simulink model "gm_uz_sine_generator_16bit"  (R2023a)
settings: Solver=FixedStepDiscrete  StartTime=0.0  StopTime=50000/100e6  RelTol=1e-3
libraries: hdlsllib x8, embmathops x8, simulink x1
(part 1 of 2)
settings Model: Creator=ts  LastModifiedBy=ts
settings SolverCC: AlgebraicLoopSolver=TrustRegion
settings DataIOCC: LimitDataPoints=on  SaveOutput=off  SaveTime=off
settings OptimizationCC: BlockReduction=off  ConditionallyExecuteInputs=off  DefaultParameterBehavior=Inlined  LifeSpan=inf
settings DebuggingCC: AlgebraicLoopMsg=error  InheritedTsInSrcMsg=none  SingleTaskRateTransMsg=error  UnconnectedInputMsg=warning  UnconnectedOutputMsg=warning  UnconnectedLineMsg=warning  AllowSymbolicDim=off  StrictBusMsg=ErrorOnBusTreatedAsVector  SFUnexpectedBacktrackingDiag=warning  SFNoUnconditionalDefaultTransitionDiag=warning  SFExecutionAtInitializationDiag=none  ArithmeticOperatorsInVariantConditions=warning
settings HardwareCC: ProdBitPerPointer=32  ProdBitPerSizeT=32  ProdBitPerPtrDiffT=32  ProdLargestAtomicFloat=None  ProdIntDivRoundTo=Undefined  ProdEndianess=Unspecified  ProdWordSize=32  ProdHWDeviceType=ASIC/FPGA->ASIC/FPGA  ProdEqTarget=off
settings ModelReferenceCC: EnableRefExpFcnMdlSchedulingChecks=on
settings SFSimCC: SimUseLocalCustomCode=off  CustomCodeUndefinedFunction=UseInterfaceOnly
settings RTWCC: RTWUseLocalCustomCode=off
settings CodeAppCC: StateflowObjectComments=on
settings GRTTargetCC: TargetLangStandard=C89/C90 (ANSI)
settings ConfigComp: CovScope=ReferencedModels  CovMetricSettings=dw  CovSaveCumulativeToWorkspaceVar=on  CovSaveSingleToWorkspaceVar=on  CovExternalEMLEnable=off  CovSFcnEnable=off

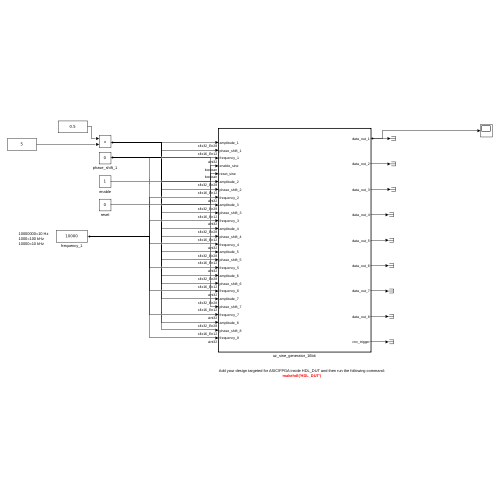
[thumbnail: Simulink's stored preview of the top-level diagram]
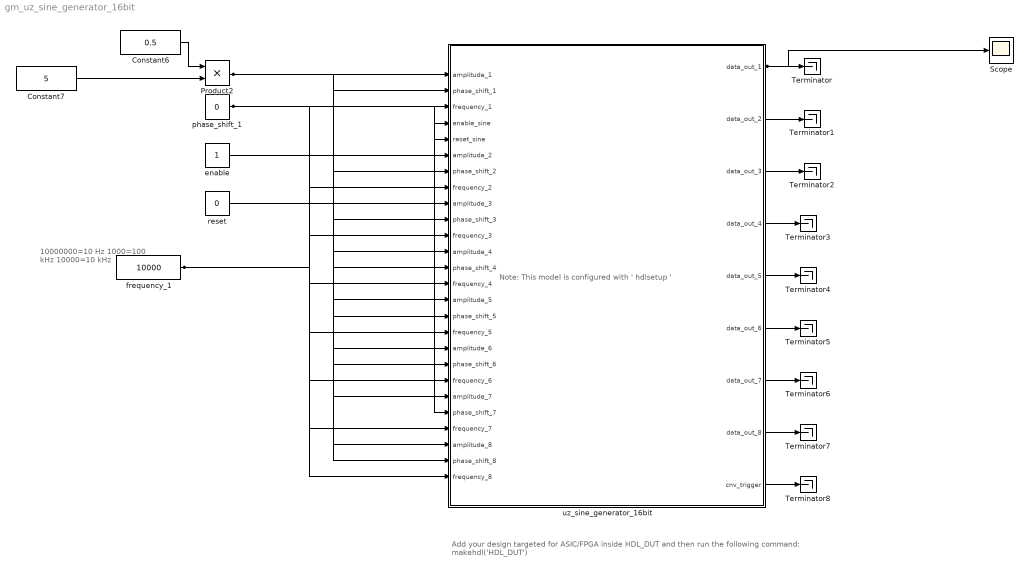
== system gm_uz_sine_generator_16bit ==
  note: 10000000=10 Hz
      | 1000=100 kHz
      | 10000=10 kHz
  note: Add your design targeted for ASIC/FPGA inside HDL_DUT and then run the following command:
      | makehdl('HDL_DUT')
  note: Note: This model is configured with ' hdlsetup '
  Constant6 : Constant  Value=0.5  SampleTime=-1
  Constant7 : Constant  Value=5  SampleTime=-1
  Product2 : Product  OutDataTypeStr=fixdt(1,32,28)
  Scope : Scope
  Terminator{,1..8} (9 alike) : Terminator
  enable : Constant  OutDataTypeStr=boolean  SampleTime=-1
  frequency_1 : Constant  Value=10000  OutDataTypeStr=uint32  SampleTime=1/100e6
  phase_shift_1 : Constant  Value=0  OutDataTypeStr=fixdt(1,16,12)  SampleTime=-1
  reset : Constant  Value=0  OutDataTypeStr=boolean  SampleTime=-1
  "uz_sine_generator_16bit " : Subsystem  TreatAsAtomicUnit=on
  wires:
  frequency_1/1 -> "uz_sine_generator_16bit "/8(frequency_2), "uz_sine_generator_16bit "/3(frequency_1), "uz_sine_generator_16bit "/11(frequency_3), "uz_sine_generator_16bit "/14(frequency_4), "uz_sine_generator_16bit "/17(frequency_5), "uz_sine_generator_16bit "/20(frequency_6), "uz_sine_generator_16bit "/23(frequency_7), "uz_sine_generator_16bit "/26(frequency_8)
  reset/1 -> "uz_sine_generator_16bit "/5(reset_sine)
  enable/1 -> "uz_sine_generator_16bit "/4(enable_sine)
  "uz_sine_generator_16bit "/9(cnv_trigger) -> Terminator8/1
  "uz_sine_generator_16bit "/8(data_out_8) -> Terminator7/1
  "uz_sine_generator_16bit "/7(data_out_7) -> Terminator6/1
  "uz_sine_generator_16bit "/6(data_out_6) -> Terminator5/1
  "uz_sine_generator_16bit "/5(data_out_5) -> Terminator4/1
  "uz_sine_generator_16bit "/4(data_out_4) -> Terminator3/1
  "uz_sine_generator_16bit "/3(data_out_3) -> Terminator2/1
  "uz_sine_generator_16bit "/2(data_out_2) -> Terminator1/1
  "uz_sine_generator_16bit "/1(data_out_1) -> Terminator/1, Scope/1
  phase_shift_1/1 -> "uz_sine_generator_16bit "/22(phase_shift_7), "uz_sine_generator_16bit "/19(phase_shift_6), "uz_sine_generator_16bit "/16(phase_shift_5), "uz_sine_generator_16bit "/10(phase_shift_3), "uz_sine_generator_16bit "/2(phase_shift_1), "uz_sine_generator_16bit "/7(phase_shift_2), "uz_sine_generator_16bit "/13(phase_shift_4), "uz_sine_generator_16bit "/25(phase_shift_8)
  Product2/1 -> "uz_sine_generator_16bit "/1(amplitude_1), "uz_sine_generator_16bit "/6(amplitude_2), "uz_sine_generator_16bit "/12(amplitude_4), "uz_sine_generator_16bit "/15(amplitude_5), "uz_sine_generator_16bit "/9(amplitude_3), "uz_sine_generator_16bit "/18(amplitude_6), "uz_sine_generator_16bit "/21(amplitude_7), "uz_sine_generator_16bit "/24(amplitude_8)
  Constant7/1 -> Product2/2
  Constant6/1 -> Product2/1

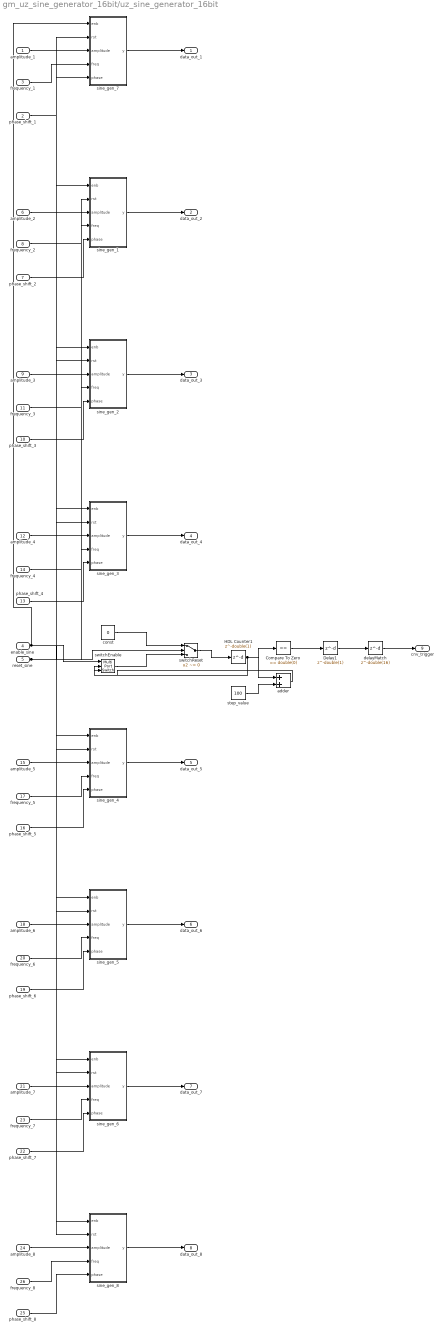
== system gm_uz_sine_generator_16bit/uz_sine_generator_16bit  ==
  amplitude_1 : Inport  OutDataTypeStr=fixdt(1, 32, 28)  PortDimensions=1  SampleTime=1e-08
  phase_shift_1 : Inport  Port=2  OutDataTypeStr=fixdt(1, 16, 12)  PortDimensions=1  SampleTime=1e-08
  frequency_1 : Inport  Port=3  OutDataTypeStr=uint32  PortDimensions=1  SampleTime=1e-08
  enable_sine : Inport  Port=4  OutDataTypeStr=boolean  PortDimensions=1  SampleTime=1e-08
  reset_sine : Inport  Port=5  OutDataTypeStr=boolean  PortDimensions=1  SampleTime=1e-08
  amplitude_2 : Inport  Port=6  OutDataTypeStr=fixdt(1, 32, 28)  PortDimensions=1  SampleTime=1e-08
  phase_shift_2 : Inport  Port=7  OutDataTypeStr=fixdt(1, 16, 12)  PortDimensions=1  SampleTime=1e-08
  frequency_2 : Inport  Port=8  OutDataTypeStr=uint32  PortDimensions=1  SampleTime=1e-08
  amplitude_3 : Inport  Port=9  OutDataTypeStr=fixdt(1, 32, 28)  PortDimensions=1  SampleTime=1e-08
  phase_shift_3 : Inport  Port=10  OutDataTypeStr=fixdt(1, 16, 12)  PortDimensions=1  SampleTime=1e-08
  frequency_3 : Inport  Port=11  OutDataTypeStr=uint32  PortDimensions=1  SampleTime=1e-08
  amplitude_4 : Inport  Port=12  OutDataTypeStr=fixdt(1, 32, 28)  PortDimensions=1  SampleTime=1e-08
  phase_shift_4 : Inport  Port=13  OutDataTypeStr=fixdt(1, 16, 12)  PortDimensions=1  SampleTime=1e-08
  frequency_4 : Inport  Port=14  OutDataTypeStr=uint32  PortDimensions=1  SampleTime=1e-08
  amplitude_5 : Inport  Port=15  OutDataTypeStr=fixdt(1, 32, 28)  PortDimensions=1  SampleTime=1e-08
  phase_shift_5 : Inport  Port=16  OutDataTypeStr=fixdt(1, 16, 12)  PortDimensions=1  SampleTime=1e-08
  frequency_5 : Inport  Port=17  OutDataTypeStr=uint32  PortDimensions=1  SampleTime=1e-08
  amplitude_6 : Inport  Port=18  OutDataTypeStr=fixdt(1, 32, 28)  PortDimensions=1  SampleTime=1e-08
  phase_shift_6 : Inport  Port=19  OutDataTypeStr=fixdt(1, 16, 12)  PortDimensions=1  SampleTime=1e-08
  frequency_6 : Inport  Port=20  OutDataTypeStr=uint32  PortDimensions=1  SampleTime=1e-08
  amplitude_7 : Inport  Port=21  OutDataTypeStr=fixdt(1, 32, 28)  PortDimensions=1  SampleTime=1e-08
  phase_shift_7 : Inport  Port=22  OutDataTypeStr=fixdt(1, 16, 12)  PortDimensions=1  SampleTime=1e-08
  frequency_7 : Inport  Port=23  OutDataTypeStr=uint32  PortDimensions=1  SampleTime=1e-08
  amplitude_8 : Inport  Port=24  OutDataTypeStr=fixdt(1, 32, 28)  PortDimensions=1  SampleTime=1e-08
  phase_shift_8 : Inport  Port=25  OutDataTypeStr=fixdt(1, 16, 12)  PortDimensions=1  SampleTime=1e-08
  frequency_8 : Inport  Port=26  OutDataTypeStr=uint32  PortDimensions=1  SampleTime=1e-08
  Compare To Zero : simulink/Logic and Bit Operations/Compare To Constant  relop===  const=double(0)  OutDataTypeStr=boolean
  Delay1 : Delay  DelayLength=double(1)  InitialCondition=0  SampleTime=1e-08
  HDL Counter1 : Delay  DelayLength=double(1)  InitialCondition=0  SampleTime=1e-08
  adder : Sum  AccumDataTypeStr=uint8  OutDataTypeStr=uint8  SampleTime=1e-08
  const : Constant  Value=0  VectorParams1D=off  OutDataTypeStr=uint8  SampleTime=1e-08
  delayMatch : Delay  DelayLength=double(16)  InitialCondition=0  SampleTime=1e-08
  sine_gen_1 : Subsystem
  sine_gen_2 : Subsystem
  sine_gen_3 : Subsystem
  sine_gen_4 : Subsystem
  sine_gen_5 : Subsystem
  sine_gen_6 : Subsystem
  sine_gen_7 : Subsystem
  sine_gen_8 : Subsystem
  step_value : Constant  Value=100  VectorParams1D=off  OutDataTypeStr=uint8  SampleTime=1e-08
  switchEnable : MultiPortSwitch  DataPortOrder=Zero-based contiguous  Inputs=2  DiagnosticForDefault=None  zeroidx=on  OutDataTypeStr=uint8  SampleTime=1e-08  SaturateOnIntegerOverflow=off  InputSameDT=off
  switchReset : Switch  Criteria=u2 ~= 0  Threshold=double(0)  OutDataTypeStr=uint8  SampleTime=1e-08  SaturateOnIntegerOverflow=off  InputSameDT=off
  data_out_1 : Outport  SampleTime=1e-08  VectorParamsAs1DForOutWhenUnconnected=off
  data_out_2 : Outport  Port=2  SampleTime=1e-08  VectorParamsAs1DForOutWhenUnconnected=off
  data_out_3 : Outport  Port=3  SampleTime=1e-08  VectorParamsAs1DForOutWhenUnconnected=off
  data_out_4 : Outport  Port=4  SampleTime=1e-08  VectorParamsAs1DForOutWhenUnconnected=off
  data_out_5 : Outport  Port=5  SampleTime=1e-08  VectorParamsAs1DForOutWhenUnconnected=off
  data_out_6 : Outport  Port=6  SampleTime=1e-08  VectorParamsAs1DForOutWhenUnconnected=off
  data_out_7 : Outport  Port=7  SampleTime=1e-08  VectorParamsAs1DForOutWhenUnconnected=off
  data_out_8 : Outport  Port=8  SampleTime=1e-08  VectorParamsAs1DForOutWhenUnconnected=off
  cnv_trigger : Outport  Port=9  SampleTime=1e-08  VectorParamsAs1DForOutWhenUnconnected=off
  wires:
  amplitude_1/1 -> sine_gen_7/3(amplitude)
  phase_shift_1/1 -> sine_gen_7/5(phase)
  frequency_1/1 -> sine_gen_7/4(freq)
  enable_sine/1 -> sine_gen_7/1(enb), sine_gen_1/1(enb), sine_gen_2/1(enb), sine_gen_3/1(enb), sine_gen_4/1(enb), sine_gen_5/1(enb), sine_gen_8/1(enb), sine_gen_6/1(enb), switchEnable/1
  reset_sine/1 -> sine_gen_1/2(rst), sine_gen_2/2(rst), sine_gen_3/2(rst), sine_gen_4/2(rst), sine_gen_5/2(rst), sine_gen_8/2(rst), sine_gen_6/2(rst), sine_gen_7/2(rst), switchReset/2
  amplitude_2/1 -> sine_gen_1/3(amplitude)
  phase_shift_2/1 -> sine_gen_1/5(phase)
  frequency_2/1 -> sine_gen_1/4(freq)
  amplitude_3/1 -> sine_gen_2/3(amplitude)
  phase_shift_3/1 -> sine_gen_2/5(phase)
  frequency_3/1 -> sine_gen_2/4(freq)
  amplitude_4/1 -> sine_gen_3/3(amplitude)
  phase_shift_4/1 -> sine_gen_3/5(phase)
  frequency_4/1 -> sine_gen_3/4(freq)
  amplitude_5/1 -> sine_gen_4/3(amplitude)
  phase_shift_5/1 -> sine_gen_4/5(phase)
  frequency_5/1 -> sine_gen_4/4(freq)
  amplitude_6/1 -> sine_gen_5/3(amplitude)
  phase_shift_6/1 -> sine_gen_5/5(phase)
  frequency_6/1 -> sine_gen_5/4(freq)
  amplitude_7/1 -> sine_gen_6/3(amplitude)
  phase_shift_7/1 -> sine_gen_6/5(phase)
  frequency_7/1 -> sine_gen_6/4(freq)
  amplitude_8/1 -> sine_gen_8/3(amplitude)
  phase_shift_8/1 -> sine_gen_8/5(phase)
  frequency_8/1 -> sine_gen_8/4(freq)
  Compare To Zero/1 -> Delay1/1
  delayMatch/1 -> cnv_trigger/1
  sine_gen_1/1(y) -> data_out_2/1
  sine_gen_7/1(y) -> data_out_1/1
  sine_gen_2/1(y) -> data_out_3/1
  sine_gen_3/1(y) -> data_out_4/1
  sine_gen_4/1(y) -> data_out_5/1
  sine_gen_5/1(y) -> data_out_6/1
  sine_gen_6/1(y) -> data_out_7/1
  sine_gen_8/1(y) -> data_out_8/1
  HDL Counter1/1 -> Compare To Zero/1, adder/1, switchEnable/2
  const/1 -> switchReset/1
  step_value/1 -> adder/2
  Delay1/1 -> delayMatch/1
  switchReset/1 -> HDL Counter1/1
  adder/1 -> switchEnable/3
  switchEnable/1 -> switchReset/3

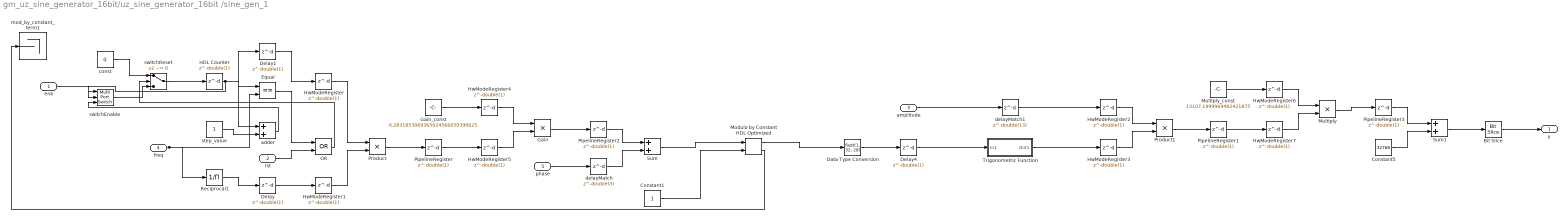
== system gm_uz_sine_generator_16bit/uz_sine_generator_16bit /sine_gen_1 ==
  enb : Inport  OutDataTypeStr=boolean  PortDimensions=1  SampleTime=1e-08
  rst : Inport  Port=2  OutDataTypeStr=boolean  PortDimensions=1  SampleTime=1e-08
  amplitude : Inport  Port=3  OutDataTypeStr=fixdt(1, 32, 28)  PortDimensions=1  SampleTime=1e-08
  freq : Inport  Port=4  OutDataTypeStr=uint32  PortDimensions=1  SampleTime=1e-08
  phase : Inport  Port=5  OutDataTypeStr=fixdt(1, 16, 12)  PortDimensions=1  SampleTime=1e-08
  Bit Slice : hdlsllib/Logic and Bit Operations/Bit Slice  lidx=double(15)  ridx=double(0)
  Constant1 : Constant  OutDataTypeStr=boolean  SampleTime=1e-08
  Constant5 : Constant  Value=32768  OutDataTypeStr=int32  SampleTime=1e-08
  Data Type Conversion : DataTypeConversion  OutDataTypeStr=fixdt(1, 32, 28)  SampleTime=1e-08  SaturateOnIntegerOverflow=off  RndMeth=Floor
  Delay : Delay  DelayLength=double(1)  InitialCondition=0  SampleTime=1e-08
  Delay1 : Delay  DelayLength=double(1)  InitialCondition=0  SampleTime=1e-08
  Delay4 : Delay  DelayLength=double(1)  InitialCondition=0  SampleTime=1e-08
  Equal : RelationalOperator  Operator===  OutDataTypeStr=boolean  SampleTime=1e-08  InputSameDT=off
  Gain : Product  Inputs=**  OutDataTypeStr=fixdt(1, 32, 28)  SampleTime=1e-08
  Gain_const : Constant  Value=6.2831853069365024566650390625  OutDataTypeStr=fixdt(0, 32, 29)  SampleTime=1e-08
  HDL Counter : Delay  DelayLength=double(1)  InitialCondition=0  SampleTime=1e-08
  HwModeRegister{,1..7} (8 alike) : Delay  DelayLength=double(1)  InitialCondition=0  SampleTime=1e-08
  Modulo by Constant HDL Optimized : embmathops/Modulo by Constant HDL Optimized  Denominator=2*pi  SimulateUsing=Code generation
      settings: LibrarySourceBlock=|
      | embeddedMatrixLib/Math Operations/Modulo by Constant
      | HDL Optimized
  Multiply : Product  Inputs=**  OutDataTypeStr=int32  SampleTime=1e-08
  Multiply_const : Constant  Value=13107.1999969482421875  OutDataTypeStr=fixdt(1, 32, 17)  SampleTime=1e-08
  OR : Logic  Operator=OR  AllPortsSameDT=off  OutDataTypeStr=boolean  SampleTime=1e-08
  PipelineRegister{,1..3} (4 alike) : Delay  DelayLength=double(1)  InitialCondition=0  SampleTime=1e-08
  Product : Product  Inputs=**  OutDataTypeStr=fixdt(0, 32, 29)  SampleTime=1e-08
  Product1 : Product  Inputs=**  OutDataTypeStr=fixdt(1, 32, 28)  SampleTime=1e-08
  Reciprocal1 : Product  Inputs=/  OutDataTypeStr=fixdt(0, 32, 31)  RndMeth=Zero  SaturateOnIntegerOverflow=on  SampleTime=1e-08
  Sum : Sum  AccumDataTypeStr=fixdt(1, 33, 28)  OutDataTypeStr=fixdt(1, 33, 28)  SampleTime=1e-08
  Sum1 : Sum  AccumDataTypeStr=int32  OutDataTypeStr=int32  SampleTime=1e-08
  Trigonometric Function : Subsystem
  adder : Sum  AccumDataTypeStr=uint32  OutDataTypeStr=uint32  SampleTime=1e-08
  const : Constant  Value=0  VectorParams1D=off  OutDataTypeStr=uint32  SampleTime=1e-08
  delayMatch : Delay  DelayLength=double(3)  InitialCondition=0  SampleTime=1e-08
  delayMatch1 : Delay  DelayLength=double(13)  InitialCondition=0  SampleTime=1e-08
  mod_by_constant_term1 : Terminator
  step_value : Constant  VectorParams1D=off  OutDataTypeStr=uint32  SampleTime=1e-08
  switchEnable : MultiPortSwitch  DataPortOrder=Zero-based contiguous  Inputs=2  DiagnosticForDefault=None  zeroidx=on  OutDataTypeStr=uint32  SampleTime=1e-08  SaturateOnIntegerOverflow=off  InputSameDT=off
  switchReset : Switch  Criteria=u2 ~= 0  Threshold=double(0)  OutDataTypeStr=uint32  SampleTime=1e-08  SaturateOnIntegerOverflow=off  InputSameDT=off
  y : Outport  SampleTime=1e-08
  wires:
  delayMatch1/1 -> HwModeRegister2/1
  delayMatch/1 -> Sum/2
  Bit Slice/1 -> y/1
  Constant1/1 -> Modulo by Constant HDL Optimized/2
  Constant5/1 -> Sum1/2
  Data Type Conversion/1 -> Delay4/1
  Delay/1 -> HwModeRegister1/1
  Delay1/1 -> HwModeRegister/1
  Sum/1 -> Modulo by Constant HDL Optimized/1
  Delay4/1 -> Trigonometric Function/1(In1)
  Trigonometric Function/1(Out1) -> HwModeRegister3/1
  PipelineRegister2/1 -> Sum/1
  Modulo by Constant HDL Optimized/1 -> Data Type Conversion/1
  Modulo by Constant HDL Optimized/2 -> mod_by_constant_term1/1
  PipelineRegister3/1 -> Sum1/1
  PipelineRegister/1 -> HwModeRegister5/1
  PipelineRegister1/1 -> HwModeRegister7/1
  Reciprocal1/1 -> Delay/1
  Sum1/1 -> Bit Slice/1
  HDL Counter/1 -> Delay1/1, Equal/1, adder/1, switchEnable/2
  const/1 -> switchReset/1
  step_value/1 -> adder/2
  Gain_const/1 -> HwModeRegister4/1
  Multiply_const/1 -> HwModeRegister6/1
  enb/1 -> switchEnable/1
  rst/1 -> OR/2
  amplitude/1 -> delayMatch1/1
  freq/1 -> Reciprocal1/1, Equal/2
  phase/1 -> delayMatch/1
  switchReset/1 -> HDL Counter/1
  adder/1 -> switchEnable/3
  switchEnable/1 -> switchReset/3
  Equal/1 -> OR/1
  OR/1 -> switchReset/2
  Product/1 -> PipelineRegister/1
  HwModeRegister/1 -> Product/1
  HwModeRegister1/1 -> Product/2
  Product1/1 -> PipelineRegister1/1
  HwModeRegister2/1 -> Product1/1
  HwModeRegister3/1 -> Product1/2
  Gain/1 -> PipelineRegister2/1
  HwModeRegister4/1 -> Gain/1
  HwModeRegister5/1 -> Gain/2
  Multiply/1 -> PipelineRegister3/1
  HwModeRegister6/1 -> Multiply/1
  HwModeRegister7/1 -> Multiply/2

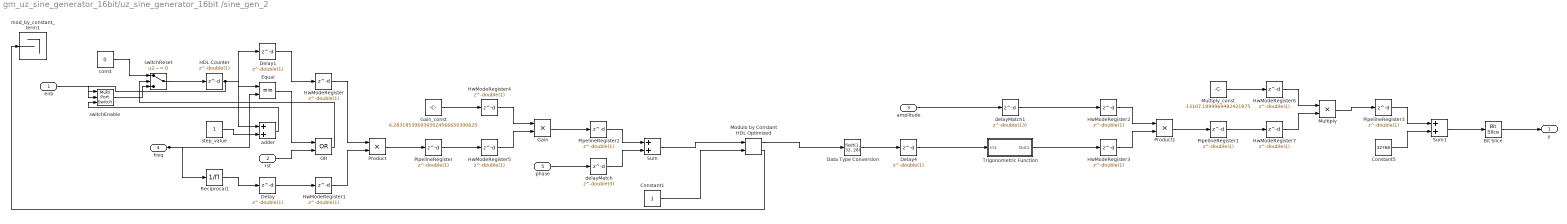
== system gm_uz_sine_generator_16bit/uz_sine_generator_16bit /sine_gen_2 ==
  enb : Inport  OutDataTypeStr=boolean  PortDimensions=1  SampleTime=1e-08
  rst : Inport  Port=2  OutDataTypeStr=boolean  PortDimensions=1  SampleTime=1e-08
  amplitude : Inport  Port=3  OutDataTypeStr=fixdt(1, 32, 28)  PortDimensions=1  SampleTime=1e-08
  freq : Inport  Port=4  OutDataTypeStr=uint32  PortDimensions=1  SampleTime=1e-08
  phase : Inport  Port=5  OutDataTypeStr=fixdt(1, 16, 12)  PortDimensions=1  SampleTime=1e-08
  Bit Slice : hdlsllib/Logic and Bit Operations/Bit Slice  lidx=double(15)  ridx=double(0)
  Constant1 : Constant  OutDataTypeStr=boolean  SampleTime=1e-08
  Constant5 : Constant  Value=32768  OutDataTypeStr=int32  SampleTime=1e-08
  Data Type Conversion : DataTypeConversion  OutDataTypeStr=fixdt(1, 32, 28)  SampleTime=1e-08  SaturateOnIntegerOverflow=off  RndMeth=Floor
  Delay : Delay  DelayLength=double(1)  InitialCondition=0  SampleTime=1e-08
  Delay1 : Delay  DelayLength=double(1)  InitialCondition=0  SampleTime=1e-08
  Delay4 : Delay  DelayLength=double(1)  InitialCondition=0  SampleTime=1e-08
  Equal : RelationalOperator  Operator===  OutDataTypeStr=boolean  SampleTime=1e-08  InputSameDT=off
  Gain : Product  Inputs=**  OutDataTypeStr=fixdt(1, 32, 28)  SampleTime=1e-08
  Gain_const : Constant  Value=6.2831853069365024566650390625  OutDataTypeStr=fixdt(0, 32, 29)  SampleTime=1e-08
  HDL Counter : Delay  DelayLength=double(1)  InitialCondition=0  SampleTime=1e-08
  HwModeRegister{,1..7} (8 alike) : Delay  DelayLength=double(1)  InitialCondition=0  SampleTime=1e-08
  Modulo by Constant HDL Optimized : embmathops/Modulo by Constant HDL Optimized  Denominator=2*pi  SimulateUsing=Code generation
      settings: LibrarySourceBlock=|
      | embeddedMatrixLib/Math Operations/Modulo by Constant
      | HDL Optimized
  Multiply : Product  Inputs=**  OutDataTypeStr=int32  SampleTime=1e-08
  Multiply_const : Constant  Value=13107.1999969482421875  OutDataTypeStr=fixdt(1, 32, 17)  SampleTime=1e-08
  OR : Logic  Operator=OR  AllPortsSameDT=off  OutDataTypeStr=boolean  SampleTime=1e-08
  PipelineRegister{,1..3} (4 alike) : Delay  DelayLength=double(1)  InitialCondition=0  SampleTime=1e-08
  Product : Product  Inputs=**  OutDataTypeStr=fixdt(0, 32, 29)  SampleTime=1e-08
  Product1 : Product  Inputs=**  OutDataTypeStr=fixdt(1, 32, 28)  SampleTime=1e-08
  Reciprocal1 : Product  Inputs=/  OutDataTypeStr=fixdt(0, 32, 31)  RndMeth=Zero  SaturateOnIntegerOverflow=on  SampleTime=1e-08
  Sum : Sum  AccumDataTypeStr=fixdt(1, 33, 28)  OutDataTypeStr=fixdt(1, 33, 28)  SampleTime=1e-08
  Sum1 : Sum  AccumDataTypeStr=int32  OutDataTypeStr=int32  SampleTime=1e-08
  Trigonometric Function : Subsystem
  adder : Sum  AccumDataTypeStr=uint32  OutDataTypeStr=uint32  SampleTime=1e-08
  const : Constant  Value=0  VectorParams1D=off  OutDataTypeStr=uint32  SampleTime=1e-08
  delayMatch : Delay  DelayLength=double(3)  InitialCondition=0  SampleTime=1e-08
  delayMatch1 : Delay  DelayLength=double(13)  InitialCondition=0  SampleTime=1e-08
  mod_by_constant_term1 : Terminator
  step_value : Constant  VectorParams1D=off  OutDataTypeStr=uint32  SampleTime=1e-08
  switchEnable : MultiPortSwitch  DataPortOrder=Zero-based contiguous  Inputs=2  DiagnosticForDefault=None  zeroidx=on  OutDataTypeStr=uint32  SampleTime=1e-08  SaturateOnIntegerOverflow=off  InputSameDT=off
  switchReset : Switch  Criteria=u2 ~= 0  Threshold=double(0)  OutDataTypeStr=uint32  SampleTime=1e-08  SaturateOnIntegerOverflow=off  InputSameDT=off
  y : Outport  SampleTime=1e-08
  wires:
  delayMatch1/1 -> HwModeRegister2/1
  delayMatch/1 -> Sum/2
  Bit Slice/1 -> y/1
  Constant1/1 -> Modulo by Constant HDL Optimized/2
  Constant5/1 -> Sum1/2
  Data Type Conversion/1 -> Delay4/1
  Delay/1 -> HwModeRegister1/1
  Delay1/1 -> HwModeRegister/1
  Sum/1 -> Modulo by Constant HDL Optimized/1
  Delay4/1 -> Trigonometric Function/1(In1)
  Trigonometric Function/1(Out1) -> HwModeRegister3/1
  PipelineRegister2/1 -> Sum/1
  Modulo by Constant HDL Optimized/1 -> Data Type Conversion/1
  Modulo by Constant HDL Optimized/2 -> mod_by_constant_term1/1
  PipelineRegister3/1 -> Sum1/1
  PipelineRegister/1 -> HwModeRegister5/1
  PipelineRegister1/1 -> HwModeRegister7/1
  Reciprocal1/1 -> Delay/1
  Sum1/1 -> Bit Slice/1
  HDL Counter/1 -> Delay1/1, Equal/1, adder/1, switchEnable/2
  const/1 -> switchReset/1
  step_value/1 -> adder/2
  Gain_const/1 -> HwModeRegister4/1
  Multiply_const/1 -> HwModeRegister6/1
  enb/1 -> switchEnable/1
  rst/1 -> OR/2
  amplitude/1 -> delayMatch1/1
  freq/1 -> Reciprocal1/1, Equal/2
  phase/1 -> delayMatch/1
  switchReset/1 -> HDL Counter/1
  adder/1 -> switchEnable/3
  switchEnable/1 -> switchReset/3
  Equal/1 -> OR/1
  OR/1 -> switchReset/2
  Product/1 -> PipelineRegister/1
  HwModeRegister/1 -> Product/1
  HwModeRegister1/1 -> Product/2
  Product1/1 -> PipelineRegister1/1
  HwModeRegister2/1 -> Product1/1
  HwModeRegister3/1 -> Product1/2
  Gain/1 -> PipelineRegister2/1
  HwModeRegister4/1 -> Gain/1
  HwModeRegister5/1 -> Gain/2
  Multiply/1 -> PipelineRegister3/1
  HwModeRegister6/1 -> Multiply/1
  HwModeRegister7/1 -> Multiply/2

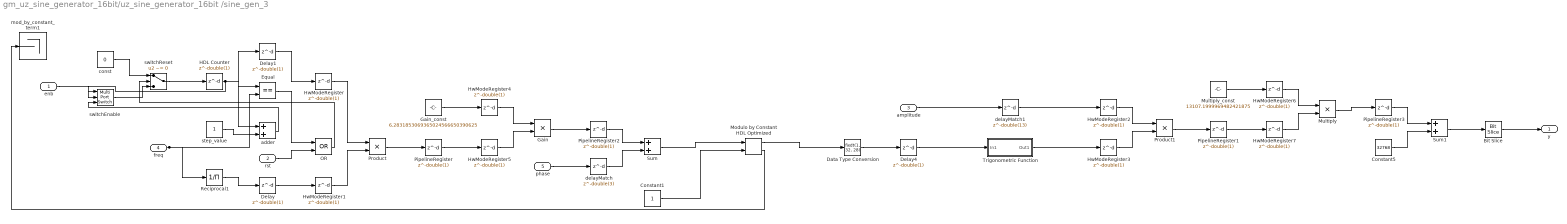
== system gm_uz_sine_generator_16bit/uz_sine_generator_16bit /sine_gen_3 ==
  enb : Inport  OutDataTypeStr=boolean  PortDimensions=1  SampleTime=1e-08
  rst : Inport  Port=2  OutDataTypeStr=boolean  PortDimensions=1  SampleTime=1e-08
  amplitude : Inport  Port=3  OutDataTypeStr=fixdt(1, 32, 28)  PortDimensions=1  SampleTime=1e-08
  freq : Inport  Port=4  OutDataTypeStr=uint32  PortDimensions=1  SampleTime=1e-08
  phase : Inport  Port=5  OutDataTypeStr=fixdt(1, 16, 12)  PortDimensions=1  SampleTime=1e-08
  Bit Slice : hdlsllib/Logic and Bit Operations/Bit Slice  lidx=double(15)  ridx=double(0)
  Constant1 : Constant  OutDataTypeStr=boolean  SampleTime=1e-08
  Constant5 : Constant  Value=32768  OutDataTypeStr=int32  SampleTime=1e-08
  Data Type Conversion : DataTypeConversion  OutDataTypeStr=fixdt(1, 32, 28)  SampleTime=1e-08  SaturateOnIntegerOverflow=off  RndMeth=Floor
  Delay : Delay  DelayLength=double(1)  InitialCondition=0  SampleTime=1e-08
  Delay1 : Delay  DelayLength=double(1)  InitialCondition=0  SampleTime=1e-08
  Delay4 : Delay  DelayLength=double(1)  InitialCondition=0  SampleTime=1e-08
  Equal : RelationalOperator  Operator===  OutDataTypeStr=boolean  SampleTime=1e-08  InputSameDT=off
  Gain : Product  Inputs=**  OutDataTypeStr=fixdt(1, 32, 28)  SampleTime=1e-08
  Gain_const : Constant  Value=6.2831853069365024566650390625  OutDataTypeStr=fixdt(0, 32, 29)  SampleTime=1e-08
  HDL Counter : Delay  DelayLength=double(1)  InitialCondition=0  SampleTime=1e-08
  HwModeRegister{,1..7} (8 alike) : Delay  DelayLength=double(1)  InitialCondition=0  SampleTime=1e-08
  Modulo by Constant HDL Optimized : embmathops/Modulo by Constant HDL Optimized  Denominator=2*pi  SimulateUsing=Code generation
      settings: LibrarySourceBlock=|
      | embeddedMatrixLib/Math Operations/Modulo by Constant
      | HDL Optimized
  Multiply : Product  Inputs=**  OutDataTypeStr=int32  SampleTime=1e-08
  Multiply_const : Constant  Value=13107.1999969482421875  OutDataTypeStr=fixdt(1, 32, 17)  SampleTime=1e-08
  OR : Logic  Operator=OR  AllPortsSameDT=off  OutDataTypeStr=boolean  SampleTime=1e-08
  PipelineRegister{,1..3} (4 alike) : Delay  DelayLength=double(1)  InitialCondition=0  SampleTime=1e-08
  Product : Product  Inputs=**  OutDataTypeStr=fixdt(0, 32, 29)  SampleTime=1e-08
  Product1 : Product  Inputs=**  OutDataTypeStr=fixdt(1, 32, 28)  SampleTime=1e-08
  Reciprocal1 : Product  Inputs=/  OutDataTypeStr=fixdt(0, 32, 31)  RndMeth=Zero  SaturateOnIntegerOverflow=on  SampleTime=1e-08
  Sum : Sum  AccumDataTypeStr=fixdt(1, 33, 28)  OutDataTypeStr=fixdt(1, 33, 28)  SampleTime=1e-08
  Sum1 : Sum  AccumDataTypeStr=int32  OutDataTypeStr=int32  SampleTime=1e-08
  Trigonometric Function : Subsystem
  adder : Sum  AccumDataTypeStr=uint32  OutDataTypeStr=uint32  SampleTime=1e-08
  const : Constant  Value=0  VectorParams1D=off  OutDataTypeStr=uint32  SampleTime=1e-08
  delayMatch : Delay  DelayLength=double(3)  InitialCondition=0  SampleTime=1e-08
  delayMatch1 : Delay  DelayLength=double(13)  InitialCondition=0  SampleTime=1e-08
  mod_by_constant_term1 : Terminator
  step_value : Constant  VectorParams1D=off  OutDataTypeStr=uint32  SampleTime=1e-08
  switchEnable : MultiPortSwitch  DataPortOrder=Zero-based contiguous  Inputs=2  DiagnosticForDefault=None  zeroidx=on  OutDataTypeStr=uint32  SampleTime=1e-08  SaturateOnIntegerOverflow=off  InputSameDT=off
  switchReset : Switch  Criteria=u2 ~= 0  Threshold=double(0)  OutDataTypeStr=uint32  SampleTime=1e-08  SaturateOnIntegerOverflow=off  InputSameDT=off
  y : Outport  SampleTime=1e-08
  wires:
  delayMatch1/1 -> HwModeRegister2/1
  delayMatch/1 -> Sum/2
  Bit Slice/1 -> y/1
  Constant1/1 -> Modulo by Constant HDL Optimized/2
  Constant5/1 -> Sum1/2
  Data Type Conversion/1 -> Delay4/1
  Delay/1 -> HwModeRegister1/1
  Delay1/1 -> HwModeRegister/1
  Sum/1 -> Modulo by Constant HDL Optimized/1
  Delay4/1 -> Trigonometric Function/1(In1)
  Trigonometric Function/1(Out1) -> HwModeRegister3/1
  PipelineRegister2/1 -> Sum/1
  Modulo by Constant HDL Optimized/1 -> Data Type Conversion/1
  Modulo by Constant HDL Optimized/2 -> mod_by_constant_term1/1
  PipelineRegister3/1 -> Sum1/1
  PipelineRegister/1 -> HwModeRegister5/1
  PipelineRegister1/1 -> HwModeRegister7/1
  Reciprocal1/1 -> Delay/1
  Sum1/1 -> Bit Slice/1
  HDL Counter/1 -> Delay1/1, Equal/1, adder/1, switchEnable/2
  const/1 -> switchReset/1
  step_value/1 -> adder/2
  Gain_const/1 -> HwModeRegister4/1
  Multiply_const/1 -> HwModeRegister6/1
  enb/1 -> switchEnable/1
  rst/1 -> OR/2
  amplitude/1 -> delayMatch1/1
  freq/1 -> Reciprocal1/1, Equal/2
  phase/1 -> delayMatch/1
  switchReset/1 -> HDL Counter/1
  adder/1 -> switchEnable/3
  switchEnable/1 -> switchReset/3
  Equal/1 -> OR/1
  OR/1 -> switchReset/2
  Product/1 -> PipelineRegister/1
  HwModeRegister/1 -> Product/1
  HwModeRegister1/1 -> Product/2
  Product1/1 -> PipelineRegister1/1
  HwModeRegister2/1 -> Product1/1
  HwModeRegister3/1 -> Product1/2
  Gain/1 -> PipelineRegister2/1
  HwModeRegister4/1 -> Gain/1
  HwModeRegister5/1 -> Gain/2
  Multiply/1 -> PipelineRegister3/1
  HwModeRegister6/1 -> Multiply/1
  HwModeRegister7/1 -> Multiply/2

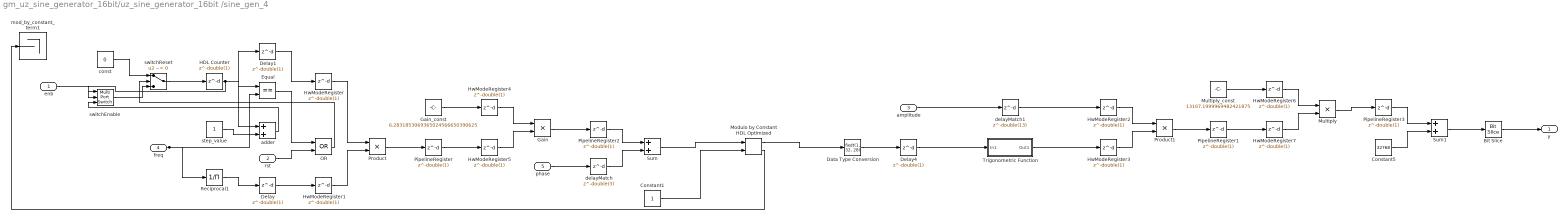
== system gm_uz_sine_generator_16bit/uz_sine_generator_16bit /sine_gen_4 ==
  enb : Inport  OutDataTypeStr=boolean  PortDimensions=1  SampleTime=1e-08
  rst : Inport  Port=2  OutDataTypeStr=boolean  PortDimensions=1  SampleTime=1e-08
  amplitude : Inport  Port=3  OutDataTypeStr=fixdt(1, 32, 28)  PortDimensions=1  SampleTime=1e-08
  freq : Inport  Port=4  OutDataTypeStr=uint32  PortDimensions=1  SampleTime=1e-08
  phase : Inport  Port=5  OutDataTypeStr=fixdt(1, 16, 12)  PortDimensions=1  SampleTime=1e-08
  Bit Slice : hdlsllib/Logic and Bit Operations/Bit Slice  lidx=double(15)  ridx=double(0)
  Constant1 : Constant  OutDataTypeStr=boolean  SampleTime=1e-08
  Constant5 : Constant  Value=32768  OutDataTypeStr=int32  SampleTime=1e-08
  Data Type Conversion : DataTypeConversion  OutDataTypeStr=fixdt(1, 32, 28)  SampleTime=1e-08  SaturateOnIntegerOverflow=off  RndMeth=Floor
  Delay : Delay  DelayLength=double(1)  InitialCondition=0  SampleTime=1e-08
  Delay1 : Delay  DelayLength=double(1)  InitialCondition=0  SampleTime=1e-08
  Delay4 : Delay  DelayLength=double(1)  InitialCondition=0  SampleTime=1e-08
  Equal : RelationalOperator  Operator===  OutDataTypeStr=boolean  SampleTime=1e-08  InputSameDT=off
  Gain : Product  Inputs=**  OutDataTypeStr=fixdt(1, 32, 28)  SampleTime=1e-08
  Gain_const : Constant  Value=6.2831853069365024566650390625  OutDataTypeStr=fixdt(0, 32, 29)  SampleTime=1e-08
  HDL Counter : Delay  DelayLength=double(1)  InitialCondition=0  SampleTime=1e-08
  HwModeRegister{,1..7} (8 alike) : Delay  DelayLength=double(1)  InitialCondition=0  SampleTime=1e-08
  Modulo by Constant HDL Optimized : embmathops/Modulo by Constant HDL Optimized  Denominator=2*pi  SimulateUsing=Code generation
      settings: LibrarySourceBlock=|
      | embeddedMatrixLib/Math Operations/Modulo by Constant
      | HDL Optimized
  Multiply : Product  Inputs=**  OutDataTypeStr=int32  SampleTime=1e-08
  Multiply_const : Constant  Value=13107.1999969482421875  OutDataTypeStr=fixdt(1, 32, 17)  SampleTime=1e-08
  OR : Logic  Operator=OR  AllPortsSameDT=off  OutDataTypeStr=boolean  SampleTime=1e-08
  PipelineRegister{,1..3} (4 alike) : Delay  DelayLength=double(1)  InitialCondition=0  SampleTime=1e-08
  Product : Product  Inputs=**  OutDataTypeStr=fixdt(0, 32, 29)  SampleTime=1e-08
  Product1 : Product  Inputs=**  OutDataTypeStr=fixdt(1, 32, 28)  SampleTime=1e-08
  Reciprocal1 : Product  Inputs=/  OutDataTypeStr=fixdt(0, 32, 31)  RndMeth=Zero  SaturateOnIntegerOverflow=on  SampleTime=1e-08
  Sum : Sum  AccumDataTypeStr=fixdt(1, 33, 28)  OutDataTypeStr=fixdt(1, 33, 28)  SampleTime=1e-08
  Sum1 : Sum  AccumDataTypeStr=int32  OutDataTypeStr=int32  SampleTime=1e-08
  Trigonometric Function : Subsystem
  adder : Sum  AccumDataTypeStr=uint32  OutDataTypeStr=uint32  SampleTime=1e-08
  const : Constant  Value=0  VectorParams1D=off  OutDataTypeStr=uint32  SampleTime=1e-08
  delayMatch : Delay  DelayLength=double(3)  InitialCondition=0  SampleTime=1e-08
  delayMatch1 : Delay  DelayLength=double(13)  InitialCondition=0  SampleTime=1e-08
  mod_by_constant_term1 : Terminator
  step_value : Constant  VectorParams1D=off  OutDataTypeStr=uint32  SampleTime=1e-08
  switchEnable : MultiPortSwitch  DataPortOrder=Zero-based contiguous  Inputs=2  DiagnosticForDefault=None  zeroidx=on  OutDataTypeStr=uint32  SampleTime=1e-08  SaturateOnIntegerOverflow=off  InputSameDT=off
  switchReset : Switch  Criteria=u2 ~= 0  Threshold=double(0)  OutDataTypeStr=uint32  SampleTime=1e-08  SaturateOnIntegerOverflow=off  InputSameDT=off
  y : Outport  SampleTime=1e-08
  wires:
  delayMatch1/1 -> HwModeRegister2/1
  delayMatch/1 -> Sum/2
  Bit Slice/1 -> y/1
  Constant1/1 -> Modulo by Constant HDL Optimized/2
  Constant5/1 -> Sum1/2
  Data Type Conversion/1 -> Delay4/1
  Delay/1 -> HwModeRegister1/1
  Delay1/1 -> HwModeRegister/1
  Sum/1 -> Modulo by Constant HDL Optimized/1
  Delay4/1 -> Trigonometric Function/1(In1)
  Trigonometric Function/1(Out1) -> HwModeRegister3/1
  PipelineRegister2/1 -> Sum/1
  Modulo by Constant HDL Optimized/1 -> Data Type Conversion/1
  Modulo by Constant HDL Optimized/2 -> mod_by_constant_term1/1
  PipelineRegister3/1 -> Sum1/1
  PipelineRegister/1 -> HwModeRegister5/1
  PipelineRegister1/1 -> HwModeRegister7/1
  Reciprocal1/1 -> Delay/1
  Sum1/1 -> Bit Slice/1
  HDL Counter/1 -> Delay1/1, Equal/1, adder/1, switchEnable/2
  const/1 -> switchReset/1
  step_value/1 -> adder/2
  Gain_const/1 -> HwModeRegister4/1
  Multiply_const/1 -> HwModeRegister6/1
  enb/1 -> switchEnable/1
  rst/1 -> OR/2
  amplitude/1 -> delayMatch1/1
  freq/1 -> Reciprocal1/1, Equal/2
  phase/1 -> delayMatch/1
  switchReset/1 -> HDL Counter/1
  adder/1 -> switchEnable/3
  switchEnable/1 -> switchReset/3
  Equal/1 -> OR/1
  OR/1 -> switchReset/2
  Product/1 -> PipelineRegister/1
  HwModeRegister/1 -> Product/1
  HwModeRegister1/1 -> Product/2
  Product1/1 -> PipelineRegister1/1
  HwModeRegister2/1 -> Product1/1
  HwModeRegister3/1 -> Product1/2
  Gain/1 -> PipelineRegister2/1
  HwModeRegister4/1 -> Gain/1
  HwModeRegister5/1 -> Gain/2
  Multiply/1 -> PipelineRegister3/1
  HwModeRegister6/1 -> Multiply/1
  HwModeRegister7/1 -> Multiply/2

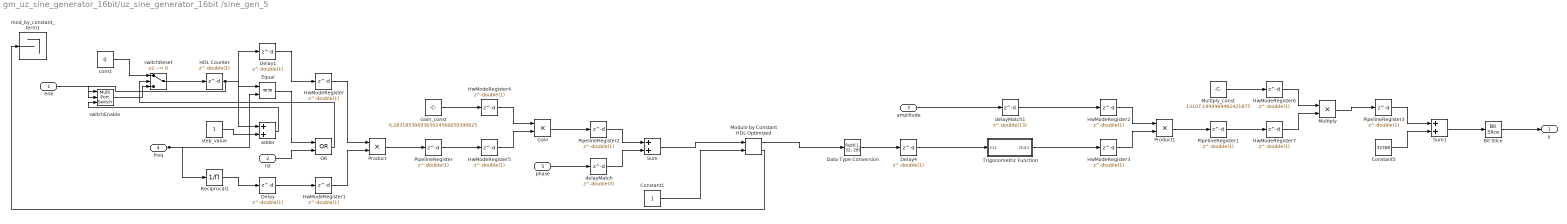
== system gm_uz_sine_generator_16bit/uz_sine_generator_16bit /sine_gen_5 ==
  enb : Inport  OutDataTypeStr=boolean  PortDimensions=1  SampleTime=1e-08
  rst : Inport  Port=2  OutDataTypeStr=boolean  PortDimensions=1  SampleTime=1e-08
  amplitude : Inport  Port=3  OutDataTypeStr=fixdt(1, 32, 28)  PortDimensions=1  SampleTime=1e-08
  freq : Inport  Port=4  OutDataTypeStr=uint32  PortDimensions=1  SampleTime=1e-08
  phase : Inport  Port=5  OutDataTypeStr=fixdt(1, 16, 12)  PortDimensions=1  SampleTime=1e-08
  Bit Slice : hdlsllib/Logic and Bit Operations/Bit Slice  lidx=double(15)  ridx=double(0)
  Constant1 : Constant  OutDataTypeStr=boolean  SampleTime=1e-08
  Constant5 : Constant  Value=32768  OutDataTypeStr=int32  SampleTime=1e-08
  Data Type Conversion : DataTypeConversion  OutDataTypeStr=fixdt(1, 32, 28)  SampleTime=1e-08  SaturateOnIntegerOverflow=off  RndMeth=Floor
  Delay : Delay  DelayLength=double(1)  InitialCondition=0  SampleTime=1e-08
  Delay1 : Delay  DelayLength=double(1)  InitialCondition=0  SampleTime=1e-08
  Delay4 : Delay  DelayLength=double(1)  InitialCondition=0  SampleTime=1e-08
  Equal : RelationalOperator  Operator===  OutDataTypeStr=boolean  SampleTime=1e-08  InputSameDT=off
  Gain : Product  Inputs=**  OutDataTypeStr=fixdt(1, 32, 28)  SampleTime=1e-08
  Gain_const : Constant  Value=6.2831853069365024566650390625  OutDataTypeStr=fixdt(0, 32, 29)  SampleTime=1e-08
  HDL Counter : Delay  DelayLength=double(1)  InitialCondition=0  SampleTime=1e-08
  HwModeRegister{,1..7} (8 alike) : Delay  DelayLength=double(1)  InitialCondition=0  SampleTime=1e-08
  Modulo by Constant HDL Optimized : embmathops/Modulo by Constant HDL Optimized  Denominator=2*pi  SimulateUsing=Code generation
      settings: LibrarySourceBlock=|
      | embeddedMatrixLib/Math Operations/Modulo by Constant
      | HDL Optimized
  Multiply : Product  Inputs=**  OutDataTypeStr=int32  SampleTime=1e-08
  Multiply_const : Constant  Value=13107.1999969482421875  OutDataTypeStr=fixdt(1, 32, 17)  SampleTime=1e-08
  OR : Logic  Operator=OR  AllPortsSameDT=off  OutDataTypeStr=boolean  SampleTime=1e-08
  PipelineRegister{,1..3} (4 alike) : Delay  DelayLength=double(1)  InitialCondition=0  SampleTime=1e-08
  Product : Product  Inputs=**  OutDataTypeStr=fixdt(0, 32, 29)  SampleTime=1e-08
  Product1 : Product  Inputs=**  OutDataTypeStr=fixdt(1, 32, 28)  SampleTime=1e-08
  Reciprocal1 : Product  Inputs=/  OutDataTypeStr=fixdt(0, 32, 31)  RndMeth=Zero  SaturateOnIntegerOverflow=on  SampleTime=1e-08
  Sum : Sum  AccumDataTypeStr=fixdt(1, 33, 28)  OutDataTypeStr=fixdt(1, 33, 28)  SampleTime=1e-08
  Sum1 : Sum  AccumDataTypeStr=int32  OutDataTypeStr=int32  SampleTime=1e-08
  Trigonometric Function : Subsystem
  adder : Sum  AccumDataTypeStr=uint32  OutDataTypeStr=uint32  SampleTime=1e-08
  const : Constant  Value=0  VectorParams1D=off  OutDataTypeStr=uint32  SampleTime=1e-08
  delayMatch : Delay  DelayLength=double(3)  InitialCondition=0  SampleTime=1e-08
  delayMatch1 : Delay  DelayLength=double(13)  InitialCondition=0  SampleTime=1e-08
  mod_by_constant_term1 : Terminator
  step_value : Constant  VectorParams1D=off  OutDataTypeStr=uint32  SampleTime=1e-08
  switchEnable : MultiPortSwitch  DataPortOrder=Zero-based contiguous  Inputs=2  DiagnosticForDefault=None  zeroidx=on  OutDataTypeStr=uint32  SampleTime=1e-08  SaturateOnIntegerOverflow=off  InputSameDT=off
  switchReset : Switch  Criteria=u2 ~= 0  Threshold=double(0)  OutDataTypeStr=uint32  SampleTime=1e-08  SaturateOnIntegerOverflow=off  InputSameDT=off
  y : Outport  SampleTime=1e-08
  wires:
  delayMatch1/1 -> HwModeRegister2/1
  delayMatch/1 -> Sum/2
  Bit Slice/1 -> y/1
  Constant1/1 -> Modulo by Constant HDL Optimized/2
  Constant5/1 -> Sum1/2
  Data Type Conversion/1 -> Delay4/1
  Delay/1 -> HwModeRegister1/1
  Delay1/1 -> HwModeRegister/1
  Sum/1 -> Modulo by Constant HDL Optimized/1
  Delay4/1 -> Trigonometric Function/1(In1)
  Trigonometric Function/1(Out1) -> HwModeRegister3/1
  PipelineRegister2/1 -> Sum/1
  Modulo by Constant HDL Optimized/1 -> Data Type Conversion/1
  Modulo by Constant HDL Optimized/2 -> mod_by_constant_term1/1
  PipelineRegister3/1 -> Sum1/1
  PipelineRegister/1 -> HwModeRegister5/1
  PipelineRegister1/1 -> HwModeRegister7/1
  Reciprocal1/1 -> Delay/1
  Sum1/1 -> Bit Slice/1
  HDL Counter/1 -> Delay1/1, Equal/1, adder/1, switchEnable/2
  const/1 -> switchReset/1
  step_value/1 -> adder/2
  Gain_const/1 -> HwModeRegister4/1
  Multiply_const/1 -> HwModeRegister6/1
  enb/1 -> switchEnable/1
  rst/1 -> OR/2
  amplitude/1 -> delayMatch1/1
  freq/1 -> Reciprocal1/1, Equal/2
  phase/1 -> delayMatch/1
  switchReset/1 -> HDL Counter/1
  adder/1 -> switchEnable/3
  switchEnable/1 -> switchReset/3
  Equal/1 -> OR/1
  OR/1 -> switchReset/2
  Product/1 -> PipelineRegister/1
  HwModeRegister/1 -> Product/1
  HwModeRegister1/1 -> Product/2
  Product1/1 -> PipelineRegister1/1
  HwModeRegister2/1 -> Product1/1
  HwModeRegister3/1 -> Product1/2
  Gain/1 -> PipelineRegister2/1
  HwModeRegister4/1 -> Gain/1
  HwModeRegister5/1 -> Gain/2
  Multiply/1 -> PipelineRegister3/1
  HwModeRegister6/1 -> Multiply/1
  HwModeRegister7/1 -> Multiply/2

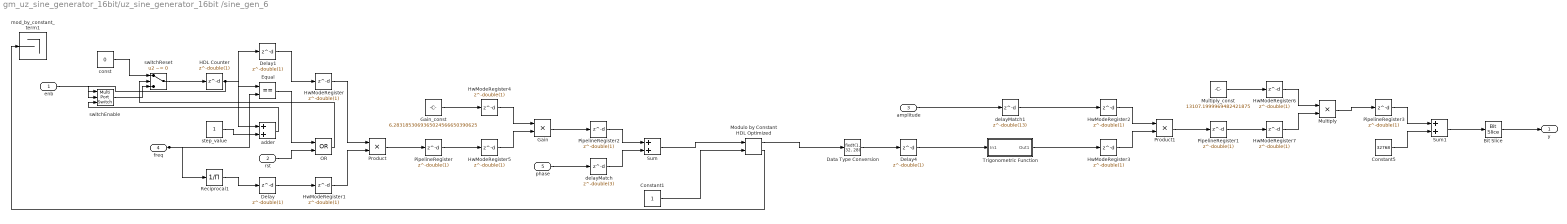
== system gm_uz_sine_generator_16bit/uz_sine_generator_16bit /sine_gen_6 ==
  enb : Inport  OutDataTypeStr=boolean  PortDimensions=1  SampleTime=1e-08
  rst : Inport  Port=2  OutDataTypeStr=boolean  PortDimensions=1  SampleTime=1e-08
  amplitude : Inport  Port=3  OutDataTypeStr=fixdt(1, 32, 28)  PortDimensions=1  SampleTime=1e-08
  freq : Inport  Port=4  OutDataTypeStr=uint32  PortDimensions=1  SampleTime=1e-08
  phase : Inport  Port=5  OutDataTypeStr=fixdt(1, 16, 12)  PortDimensions=1  SampleTime=1e-08
  Bit Slice : hdlsllib/Logic and Bit Operations/Bit Slice  lidx=double(15)  ridx=double(0)
  Constant1 : Constant  OutDataTypeStr=boolean  SampleTime=1e-08
  Constant5 : Constant  Value=32768  OutDataTypeStr=int32  SampleTime=1e-08
  Data Type Conversion : DataTypeConversion  OutDataTypeStr=fixdt(1, 32, 28)  SampleTime=1e-08  SaturateOnIntegerOverflow=off  RndMeth=Floor
  Delay : Delay  DelayLength=double(1)  InitialCondition=0  SampleTime=1e-08
  Delay1 : Delay  DelayLength=double(1)  InitialCondition=0  SampleTime=1e-08
  Delay4 : Delay  DelayLength=double(1)  InitialCondition=0  SampleTime=1e-08
  Equal : RelationalOperator  Operator===  OutDataTypeStr=boolean  SampleTime=1e-08  InputSameDT=off
  Gain : Product  Inputs=**  OutDataTypeStr=fixdt(1, 32, 28)  SampleTime=1e-08
  Gain_const : Constant  Value=6.2831853069365024566650390625  OutDataTypeStr=fixdt(0, 32, 29)  SampleTime=1e-08
  HDL Counter : Delay  DelayLength=double(1)  InitialCondition=0  SampleTime=1e-08
  HwModeRegister{,1..7} (8 alike) : Delay  DelayLength=double(1)  InitialCondition=0  SampleTime=1e-08
  Modulo by Constant HDL Optimized : embmathops/Modulo by Constant HDL Optimized  Denominator=2*pi  SimulateUsing=Code generation
      settings: LibrarySourceBlock=|
      | embeddedMatrixLib/Math Operations/Modulo by Constant
      | HDL Optimized
  Multiply : Product  Inputs=**  OutDataTypeStr=int32  SampleTime=1e-08
  Multiply_const : Constant  Value=13107.1999969482421875  OutDataTypeStr=fixdt(1, 32, 17)  SampleTime=1e-08
  OR : Logic  Operator=OR  AllPortsSameDT=off  OutDataTypeStr=boolean  SampleTime=1e-08
  PipelineRegister{,1..3} (4 alike) : Delay  DelayLength=double(1)  InitialCondition=0  SampleTime=1e-08
  Product : Product  Inputs=**  OutDataTypeStr=fixdt(0, 32, 29)  SampleTime=1e-08
  Product1 : Product  Inputs=**  OutDataTypeStr=fixdt(1, 32, 28)  SampleTime=1e-08
  Reciprocal1 : Product  Inputs=/  OutDataTypeStr=fixdt(0, 32, 31)  RndMeth=Zero  SaturateOnIntegerOverflow=on  SampleTime=1e-08
  Sum : Sum  AccumDataTypeStr=fixdt(1, 33, 28)  OutDataTypeStr=fixdt(1, 33, 28)  SampleTime=1e-08
  Sum1 : Sum  AccumDataTypeStr=int32  OutDataTypeStr=int32  SampleTime=1e-08
  Trigonometric Function : Subsystem
  adder : Sum  AccumDataTypeStr=uint32  OutDataTypeStr=uint32  SampleTime=1e-08
  const : Constant  Value=0  VectorParams1D=off  OutDataTypeStr=uint32  SampleTime=1e-08
  delayMatch : Delay  DelayLength=double(3)  InitialCondition=0  SampleTime=1e-08
  delayMatch1 : Delay  DelayLength=double(13)  InitialCondition=0  SampleTime=1e-08
  mod_by_constant_term1 : Terminator
  step_value : Constant  VectorParams1D=off  OutDataTypeStr=uint32  SampleTime=1e-08
  switchEnable : MultiPortSwitch  DataPortOrder=Zero-based contiguous  Inputs=2  DiagnosticForDefault=None  zeroidx=on  OutDataTypeStr=uint32  SampleTime=1e-08  SaturateOnIntegerOverflow=off  InputSameDT=off
  switchReset : Switch  Criteria=u2 ~= 0  Threshold=double(0)  OutDataTypeStr=uint32  SampleTime=1e-08  SaturateOnIntegerOverflow=off  InputSameDT=off
  y : Outport  SampleTime=1e-08
  wires:
  delayMatch1/1 -> HwModeRegister2/1
  delayMatch/1 -> Sum/2
  Bit Slice/1 -> y/1
  Constant1/1 -> Modulo by Constant HDL Optimized/2
  Constant5/1 -> Sum1/2
  Data Type Conversion/1 -> Delay4/1
  Delay/1 -> HwModeRegister1/1
  Delay1/1 -> HwModeRegister/1
  Sum/1 -> Modulo by Constant HDL Optimized/1
  Delay4/1 -> Trigonometric Function/1(In1)
  Trigonometric Function/1(Out1) -> HwModeRegister3/1
  PipelineRegister2/1 -> Sum/1
  Modulo by Constant HDL Optimized/1 -> Data Type Conversion/1
  Modulo by Constant HDL Optimized/2 -> mod_by_constant_term1/1
  PipelineRegister3/1 -> Sum1/1
  PipelineRegister/1 -> HwModeRegister5/1
  PipelineRegister1/1 -> HwModeRegister7/1
  Reciprocal1/1 -> Delay/1
  Sum1/1 -> Bit Slice/1
  HDL Counter/1 -> Delay1/1, Equal/1, adder/1, switchEnable/2
  const/1 -> switchReset/1
  step_value/1 -> adder/2
  Gain_const/1 -> HwModeRegister4/1
  Multiply_const/1 -> HwModeRegister6/1
  enb/1 -> switchEnable/1
  rst/1 -> OR/2
  amplitude/1 -> delayMatch1/1
  freq/1 -> Reciprocal1/1, Equal/2
  phase/1 -> delayMatch/1
  switchReset/1 -> HDL Counter/1
  adder/1 -> switchEnable/3
  switchEnable/1 -> switchReset/3
  Equal/1 -> OR/1
  OR/1 -> switchReset/2
  Product/1 -> PipelineRegister/1
  HwModeRegister/1 -> Product/1
  HwModeRegister1/1 -> Product/2
  Product1/1 -> PipelineRegister1/1
  HwModeRegister2/1 -> Product1/1
  HwModeRegister3/1 -> Product1/2
  Gain/1 -> PipelineRegister2/1
  HwModeRegister4/1 -> Gain/1
  HwModeRegister5/1 -> Gain/2
  Multiply/1 -> PipelineRegister3/1
  HwModeRegister6/1 -> Multiply/1
  HwModeRegister7/1 -> Multiply/2

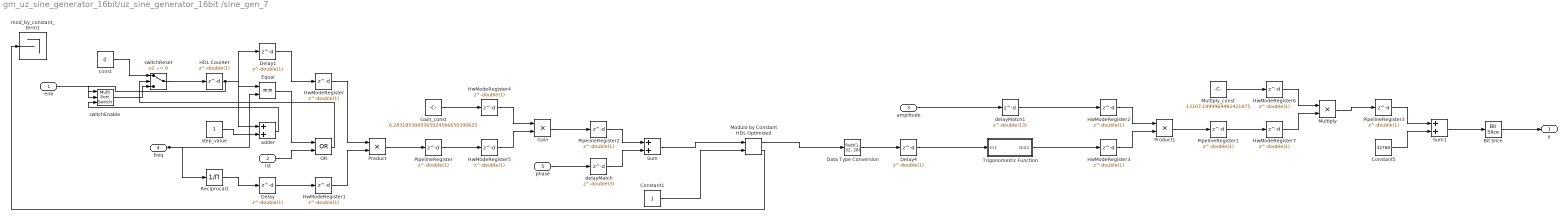
== system gm_uz_sine_generator_16bit/uz_sine_generator_16bit /sine_gen_7 ==
  enb : Inport  OutDataTypeStr=boolean  PortDimensions=1  SampleTime=1e-08
  rst : Inport  Port=2  OutDataTypeStr=boolean  PortDimensions=1  SampleTime=1e-08
  amplitude : Inport  Port=3  OutDataTypeStr=fixdt(1, 32, 28)  PortDimensions=1  SampleTime=1e-08
  freq : Inport  Port=4  OutDataTypeStr=uint32  PortDimensions=1  SampleTime=1e-08
  phase : Inport  Port=5  OutDataTypeStr=fixdt(1, 16, 12)  PortDimensions=1  SampleTime=1e-08
  Bit Slice : hdlsllib/Logic and Bit Operations/Bit Slice  lidx=double(15)  ridx=double(0)
  Constant1 : Constant  OutDataTypeStr=boolean  SampleTime=1e-08
  Constant5 : Constant  Value=32768  OutDataTypeStr=int32  SampleTime=1e-08
  Data Type Conversion : DataTypeConversion  OutDataTypeStr=fixdt(1, 32, 28)  SampleTime=1e-08  SaturateOnIntegerOverflow=off  RndMeth=Floor
  Delay : Delay  DelayLength=double(1)  InitialCondition=0  SampleTime=1e-08
  Delay1 : Delay  DelayLength=double(1)  InitialCondition=0  SampleTime=1e-08
  Delay4 : Delay  DelayLength=double(1)  InitialCondition=0  SampleTime=1e-08
  Equal : RelationalOperator  Operator===  OutDataTypeStr=boolean  SampleTime=1e-08  InputSameDT=off
  Gain : Product  Inputs=**  OutDataTypeStr=fixdt(1, 32, 28)  SampleTime=1e-08
  Gain_const : Constant  Value=6.2831853069365024566650390625  OutDataTypeStr=fixdt(0, 32, 29)  SampleTime=1e-08
  HDL Counter : Delay  DelayLength=double(1)  InitialCondition=0  SampleTime=1e-08
  HwModeRegister{,1..7} (8 alike) : Delay  DelayLength=double(1)  InitialCondition=0  SampleTime=1e-08
  Modulo by Constant HDL Optimized : embmathops/Modulo by Constant HDL Optimized  Denominator=2*pi  SimulateUsing=Code generation
      settings: LibrarySourceBlock=|
      | embeddedMatrixLib/Math Operations/Modulo by Constant
      | HDL Optimized
  Multiply : Product  Inputs=**  OutDataTypeStr=int32  SampleTime=1e-08
  Multiply_const : Constant  Value=13107.1999969482421875  OutDataTypeStr=fixdt(1, 32, 17)  SampleTime=1e-08
  OR : Logic  Operator=OR  AllPortsSameDT=off  OutDataTypeStr=boolean  SampleTime=1e-08
  PipelineRegister{,1..3} (4 alike) : Delay  DelayLength=double(1)  InitialCondition=0  SampleTime=1e-08
  Product : Product  Inputs=**  OutDataTypeStr=fixdt(0, 32, 29)  SampleTime=1e-08
  Product1 : Product  Inputs=**  OutDataTypeStr=fixdt(1, 32, 28)  SampleTime=1e-08
  Reciprocal1 : Product  Inputs=/  OutDataTypeStr=fixdt(0, 32, 31)  RndMeth=Zero  SaturateOnIntegerOverflow=on  SampleTime=1e-08
  Sum : Sum  AccumDataTypeStr=fixdt(1, 33, 28)  OutDataTypeStr=fixdt(1, 33, 28)  SampleTime=1e-08
  Sum1 : Sum  AccumDataTypeStr=int32  OutDataTypeStr=int32  SampleTime=1e-08
  Trigonometric Function : Subsystem
  adder : Sum  AccumDataTypeStr=uint32  OutDataTypeStr=uint32  SampleTime=1e-08
  const : Constant  Value=0  VectorParams1D=off  OutDataTypeStr=uint32  SampleTime=1e-08
  delayMatch : Delay  DelayLength=double(3)  InitialCondition=0  SampleTime=1e-08
  delayMatch1 : Delay  DelayLength=double(13)  InitialCondition=0  SampleTime=1e-08
  mod_by_constant_term1 : Terminator
  step_value : Constant  VectorParams1D=off  OutDataTypeStr=uint32  SampleTime=1e-08
  switchEnable : MultiPortSwitch  DataPortOrder=Zero-based contiguous  Inputs=2  DiagnosticForDefault=None  zeroidx=on  OutDataTypeStr=uint32  SampleTime=1e-08  SaturateOnIntegerOverflow=off  InputSameDT=off
  switchReset : Switch  Criteria=u2 ~= 0  Threshold=double(0)  OutDataTypeStr=uint32  SampleTime=1e-08  SaturateOnIntegerOverflow=off  InputSameDT=off
  y : Outport  SampleTime=1e-08
  wires:
  delayMatch1/1 -> HwModeRegister2/1
  delayMatch/1 -> Sum/2
  Bit Slice/1 -> y/1
  Constant1/1 -> Modulo by Constant HDL Optimized/2
  Constant5/1 -> Sum1/2
  Data Type Conversion/1 -> Delay4/1
  Delay/1 -> HwModeRegister1/1
  Delay1/1 -> HwModeRegister/1
  Sum/1 -> Modulo by Constant HDL Optimized/1
  Delay4/1 -> Trigonometric Function/1(In1)
  Trigonometric Function/1(Out1) -> HwModeRegister3/1
  PipelineRegister2/1 -> Sum/1
  Modulo by Constant HDL Optimized/1 -> Data Type Conversion/1
  Modulo by Constant HDL Optimized/2 -> mod_by_constant_term1/1
  PipelineRegister3/1 -> Sum1/1
  PipelineRegister/1 -> HwModeRegister5/1
  PipelineRegister1/1 -> HwModeRegister7/1
  Reciprocal1/1 -> Delay/1
  Sum1/1 -> Bit Slice/1
  HDL Counter/1 -> Delay1/1, Equal/1, adder/1, switchEnable/2
  const/1 -> switchReset/1
  step_value/1 -> adder/2
  Gain_const/1 -> HwModeRegister4/1
  Multiply_const/1 -> HwModeRegister6/1
  enb/1 -> switchEnable/1
  rst/1 -> OR/2
  amplitude/1 -> delayMatch1/1
  freq/1 -> Reciprocal1/1, Equal/2
  phase/1 -> delayMatch/1
  switchReset/1 -> HDL Counter/1
  adder/1 -> switchEnable/3
  switchEnable/1 -> switchReset/3
  Equal/1 -> OR/1
  OR/1 -> switchReset/2
  Product/1 -> PipelineRegister/1
  HwModeRegister/1 -> Product/1
  HwModeRegister1/1 -> Product/2
  Product1/1 -> PipelineRegister1/1
  HwModeRegister2/1 -> Product1/1
  HwModeRegister3/1 -> Product1/2
  Gain/1 -> PipelineRegister2/1
  HwModeRegister4/1 -> Gain/1
  HwModeRegister5/1 -> Gain/2
  Multiply/1 -> PipelineRegister3/1
  HwModeRegister6/1 -> Multiply/1
  HwModeRegister7/1 -> Multiply/2
